simulink model "EDriveAddTask1"  (R2021b)
settings: Solver=ode23t  StartTime=0.0  StopTime=1  MaxStep=2e-5  RelTol=1e-3
values from neighbouring files (symbols this model uses):
  J_motor = 0.000610871894223    [var_10.mat]
  L_phase = 0.00332259990587    [var_10.mat]
  M_nom = 0.61236365542    [var_10.mat]
  psi = 0.0961787034043    [var_10.mat]
  R_phase = 0.753894801324    [var_10.mat]
  U_nom = 48    [var_10.mat]
undefined symbols (not defined in the file or in its folder): Ki_i, Ki_w, Kp_i, Kp_w, w_z
libraries: simulink x1
settings Model: Creator=Denis  LastModifiedBy=Denis

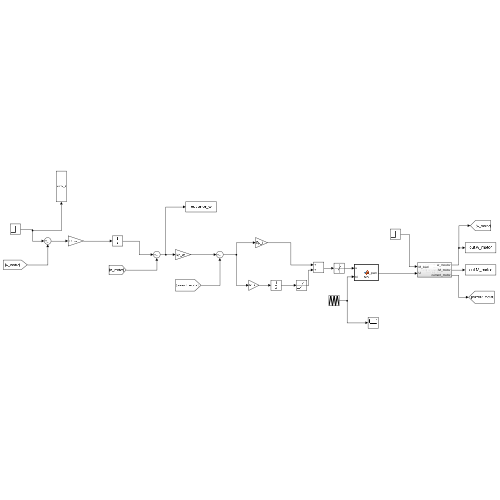
[thumbnail: Simulink's stored preview of the top-level diagram]
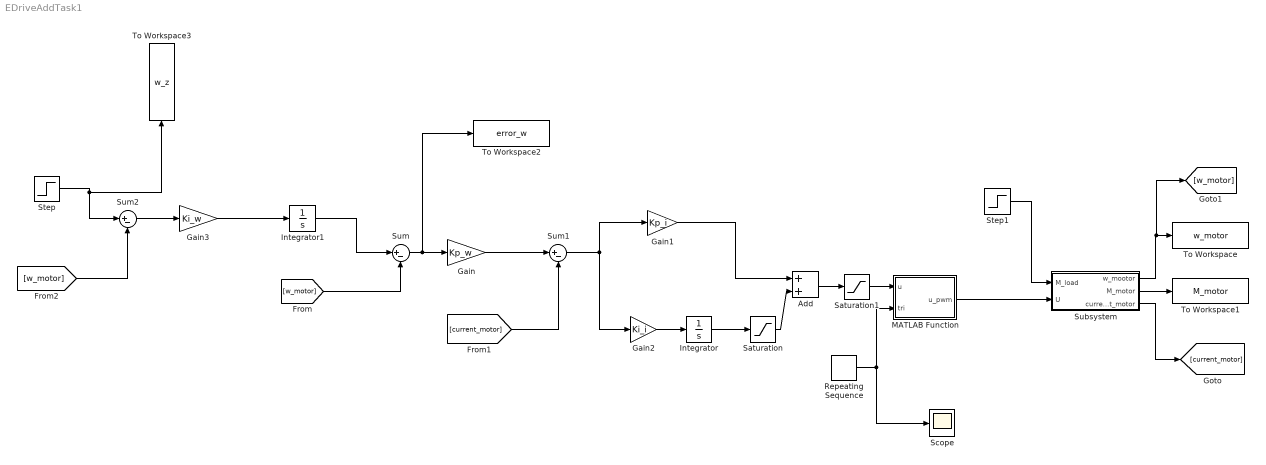
== system EDriveAddTask1 ==
  Add : Sum
  Gain : Gain  Gain=Kp_w
  Gain1 : Gain  Gain=Kp_i
  Gain2 : Gain  Gain=Ki_i
  Gain3 : Gain  Gain=Ki_w
  Integrator : Integrator
  Integrator1 : Integrator
  MATLAB Function : MATLAB Function  TreatAsAtomicUnit=on
  Repeating Sequence : simulink/Sources/Repeating Sequence  rep_seq_t=[0 1/10000 1/5000]  rep_seq_y=[-1 1 -1]
  Saturation : Saturate  UpperLimit=1  LowerLimit=-1
  Saturation1 : Saturate  UpperLimit=1  LowerLimit=-1
  Scope : Scope
  Step : Step  Time=0.5  After=w_z  SampleTime=0
  Step1 : Step  Time=0  Before=M_nom  After=M_nom  SampleTime=0
  Subsystem : Subsystem
  Sum : Sum  Inputs=|+-
  Sum1 : Sum  Inputs=|+-
  Sum2 : Sum  Inputs=|+-
  To Workspace : ToWorkspace  VariableName=w_motor  SaveFormat=Timeseries  SampleTime=-1
  To Workspace1 : ToWorkspace  VariableName=M_motor  SaveFormat=Timeseries  SampleTime=-1
  To Workspace2 : ToWorkspace  VariableName=error_w  SaveFormat=Timeseries  SampleTime=-1
  To Workspace3 : ToWorkspace  VariableName=w_z  SaveFormat=Timeseries  SampleTime=-1
  wires:
  Integrator1/1 -> Sum/1
  Step/1 -> To Workspace3/1, Sum2/1
  [w_motor] -> Sum2/2
  Sum2/1 -> Gain3/1
  Add/1 -> Saturation1/1
  Subsystem/1(w_mootor) -> [w_motor], To Workspace/1
  [w_motor] -> Sum/2
  Gain1/1 -> Add/1
  Sum1/1 -> Gain1/1, Gain2/1
  Sum/1 -> To Workspace2/1, Gain/1
  Gain/1 -> Sum1/1
  Subsystem/3(current_motor) -> [current_motor]
  Saturation/1 -> Add/2
  [current_motor] -> Sum1/2
  Gain2/1 -> Integrator/1
  Gain3/1 -> Integrator1/1
  Subsystem/2(M_motor) -> To Workspace1/1
  Step1/1 -> Subsystem/1(M_load)
  Integrator/1 -> Saturation/1
  Saturation1/1 -> MATLAB Function/1(u)
  Repeating Sequence/1 -> Scope/1, MATLAB Function/2(tri)
  MATLAB Function/1(u_pwm) -> Subsystem/2(U)

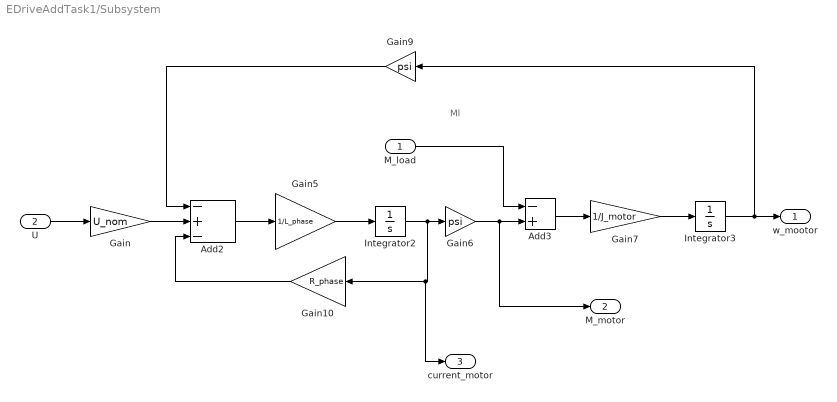
== system EDriveAddTask1/Subsystem ==
  note: Ml
  M_load : Inport
  U : Inport  Port=2
  Add2 : Sum  Inputs=-+-
  Add3 : Sum  Inputs=-+
  Gain : Gain  Gain=U_nom
  Gain10 : Gain  Gain=R_phase
  Gain5 : Gain  Gain=1/L_phase
  Gain6 : Gain  Gain=psi
  Gain7 : Gain  Gain=1/J_motor
  Gain9 : Gain  Gain=psi
  Integrator2 : Integrator
  Integrator3 : Integrator
  w_mootor : Outport
  M_motor : Outport  Port=2
  current_motor : Outport  Port=3
  wires:
  Integrator2/1 -> current_motor/1, Gain10/1, Gain6/1
  Add2/1 -> Gain5/1
  Gain/1 -> Add2/2
  Gain5/1 -> Integrator2/1
  Gain9/1 -> Add2/1
  U/1 -> Gain/1
  Gain7/1 -> Integrator3/1
  Add3/1 -> Gain7/1
  Gain6/1 -> M_motor/1, Add3/2
  M_load/1 -> Add3/1
  Gain10/1 -> Add2/3
  Integrator3/1 -> w_mootor/1, Gain9/1

== matlab function EDriveAddTask1/MATLAB Function ==
  data: u input; u_pwm output; tri input
function u_pwm = fcn(u, tri)
if u>=tri
    u_pwm = 1;
else
    u_pwm = -1;
end
